simulink model "gm_RRCFilter"  (R2023b)
settings: Solver=FixedStepAuto  StartTime=0.0  StopTime=100.0  RelTol=1e-3  EnableMultiTasking=on
libraries: dspmlti4 x1, dspsrcs4 x1
settings Model: Creator=31651  LastModifiedBy=31651
settings SolverCC: PositivePriorityOrder=on
settings OptimizationCC: BlockReduction=off  ConditionallyExecuteInputs=off  EnhancedBackFolding=on  PassReuseOutputArgsAs=Individual arguments  ZeroExternalMemoryAtStartup=off  ZeroInternalMemoryAtStartup=off  MaxStackSize=64  OptimizeBlockOrder=speed  DifferentSizesBufferReuse=on  OptimizationCustomize=off  EfficientTunableParamExpr=on
settings DebuggingCC: InheritedTsInSrcMsg=none  SingleTaskRateTransMsg=error  ParameterPrecisionLossMsg=none  ParameterTunabilityLossMsg=error
settings HardwareCC: ProdBitPerPointer=32  ProdBitPerSizeT=32  ProdBitPerPtrDiffT=32  ProdLargestAtomicInteger=Long  ProdLargestAtomicFloat=Double  ProdWordSize=32  ProdHWDeviceType=ARM Compatible->ARM Cortex  HardwareBoardFeatureSet=SoCBlockset
settings ModelReferenceCC: ModelReferenceNumInstancesAllowed=Single
settings SFSimCC: MATLABDynamicMemAlloc=off
settings RTWCC: Description=Embedded Coder  SystemTargetFile=ert.tlc  HardwareBoard=ZedBoard  TLCOptions="-aInlineSetEventsForThisBaseRateFcn=TLC_FALSE -aSuppressMultiTaskScheduler=TLC_FALSE  -aRateBasedStepFcn=0"  TemplateMakefile=ert_default_tmf
settings CodeAppCC: ForceParamTrailComments=on  IgnoreCustomStorageClasses=off  OperatorAnnotations=on  SimulinkDataObjDesc=on  SFDataObjDesc=on  InsertBlockDesc=on

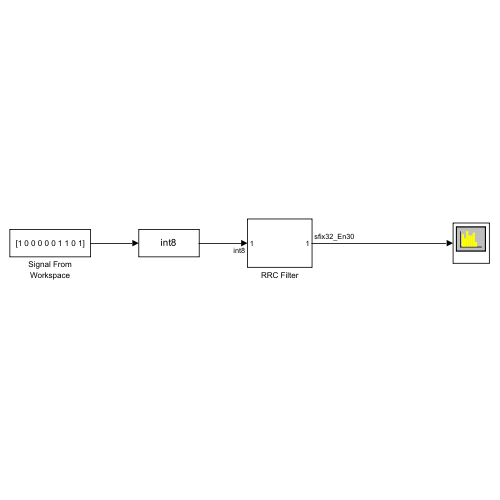
[thumbnail: Simulink's stored preview of the top-level diagram]
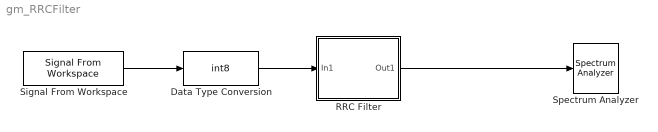
== system gm_RRCFilter ==
  Data Type Conversion : DataTypeConversion  OutDataTypeStr=int8  SaturateOnIntegerOverflow=off  RndMeth=Floor
  RRC Filter : Subsystem
  Signal From Workspace : dspsrcs4/Signal From Workspace  X=[1 0 0 0 0 0 1 1 0 1]  Ts=1  nsamps=1  OutputAfterFinalValue=Setting to zero  ignoreOrWarnInputAndFrameLengths=off  OutputFrames=off
  Spectrum Analyzer : SpectrumAnalyzer  WindowPosition=[560.000000,290.000000,800.000000,500.000000,]  Visible=on  ScopeFrameLocation=window  YLimits=[-1,1]
      settings: OpenAtSimulationStart=off
  wires:
  Data Type Conversion/1 -> RRC Filter/1(In1)
  RRC Filter/1(Out1) -> Spectrum Analyzer/1
  Signal From Workspace/1 -> Data Type Conversion/1

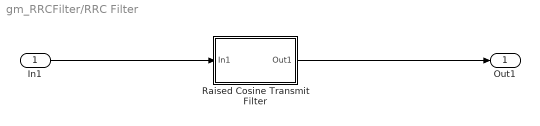
== system gm_RRCFilter/RRC Filter ==
  In1 : Inport  OutDataTypeStr=int8  PortDimensions=1  SampleTime=1
  Raised Cosine Transmit Filter : Subsystem  mask(Raised Cosine Transmit Filter){filtType=Square root, R=double(0.35), filtSpan=double(10), N=double(8), filterGain=double(1), InputProcessing=Elements as channels (sample based), RateOptions=Allow multirate processing, framing=Mute, checkCoeff=on, variableName=reshape(double([0.0026527855208223674 0.0011289546396784642 -0.0008407326480319395 -0.00276367829210128 -0.004110944765368385 -0.004461362499463928 -0.003631504382928873 -0.001754140268900142 0.0007223681197420734 0.0031229931857521803 0.004709784599647098 0.004885171607650034 0.0033846054323965124 0.0004047716742814459 -0.0033763672523499932 -0.006908879439330136 -0.00899992193184229 -0.008620760449754293 -0.005224208699525725 0.0010072932270158315 0.009056961535619827 0.01716189202348441 0.023104501384526945 0.024670913641949364 0.020196270831997543 0.009086336159429796 -0.007804452542466291 -0.028041986077568522 -0.047791391302472425 -0.06231040781338443 -0.06669696670055805 -0.056772614240839 -0.02994482367854878 0.014118459714553666 0.07314561775450068 0.14233999357591096 0.21489687901792265 0.2828943370509198 0.33842104994516803 0.37475541159859566 0.38739472380436457 0.37475541159859566 0.33842104994516803 0.2828943370509198 0.21489687901792265 0.14233999357591096 0.07314561775450068 0.014118459714553666 -0.02994482367854878 -0.056772614240839 -0.06669696670055805 -0.06231040781338443 -0.047791391302472425 -0.028041986077568522 -0.007804452542466291 0.009086336159429796 0.020196270831997543 0.024670913641949364 0.023104501384526945 0.01716189202348441 0.009056961535619827 0.0010072932270158315 -0.005224208699525725 -0.008620760449754293 -0.00899992193184229 -0.006908879439330136 -0.0033763672523499932 0.0004047716742814459 0.0033846054323965124 0.004885171607650034 0.004709784599647098 0.0031229931857521803 0.0007223681197420734 -0.001754140268900142 -0.003631504382928873 -0.004461362499463928 -0.004110944765368385 -0.00276367829210128 -0.0008407326480319395 0.0011289546396784642 0.0026527855208223674]).', [1  81]), checkGain=Normalized, sampMode=Mute, saveAsFlag=double(0), currentFiltSpan=double(10), D=double(5), launchFVT=on, roundingMode=Floor, overflowMode=off, coeffMode=Binary point scaling, coeffWordLength=double(32), coeffFracLength=double(30), coeffDataTypeStr=fixdt(1,32,30), coeffMin=[], coeffMax=[], coeffLastDataTypeStr=fixdt(1,32,30), prodOutputMode=Binary point scaling, prodOutputWordLength=double(32), prodOutputFracLength=double(30), prodOutputDataTypeStr=fixdt(1,32,30), prodOutputLastDataTypeStr=fixdt(1,32,30), accumMode=Binary point scaling, accumWordLength=double(32), accumFracLength=double(30), accumDataTypeStr=fixdt(1,32,30), accumLastDataTypeStr=fixdt(1,32,30), outputMode=Binary point scaling, outputWordLength=double(32), outputFracLength=double(30), outputDataTypeStr=fixdt(1,32,30), outputMin=[], outputMax=[], outputLastDataTypeStr=fixdt(1,32,30), LockScale=on}
      mask prompts: filtType "Filter shape:"; R "Rolloff factor:"; filtSpan "Filter span in symbols:"; N "Output samples per symbol:"; filterGain "Linear amplitude filter gain:"; InputProcessing "dsp:FIRMultirateBlockDialog:InputProc_MP"; RateOptions "dsp:FIRMultirateBlockDialog:RateOptions_MP"; checkCoeff "Export filter coefficients to workspace"; variableName "Coefficient variable name:"; checkGain "Filter gain:"; sampMode "Input sampling mode:"; saveAsFlag "Save_as flag:"; currentFiltSpan "Current filter span in symbols:"; D "Group delay (number of symbols):"; launchFVT "Visualize filter with FVTool"; roundingMode "dspshared:FixptDialog:roundingMode"; overflowMode "Simulink:masks:SaturateOnIntegerOverflow_MP"; LockScale "dspshared:FixptDialog:lockAgnstChanges"
      mask help: Upsample and filter the input signal using a normal or square root raised cosine FIR filter.
      mask init:
      | D = double(5);
      | InputProcessing = double(2);
      | LockScale = double(1);
      | N = double(8);
      | R = double(0.35);
      | RateOptions = double(2);
      | accumDataTypeStr = fixdt(1,32,30);
      | accumFracLength = double(30);
      | accumLastDataTypeStr = 'fixdt(1,32,30)';
      | accumMode = double(4);
      | accumWordLength = double(32);
      | checkCoeff = double(1);
      | checkGain = double(1);
      | coeff = reshape(double([0.0026527855208223674 0.0011289546396784642 -0.0008407326480319395 -0.00276367829210128 -0.004110944765368385 -0.004461362499463928 -0.003631504382928873 -0.001754140268900142 0.0007223681197420734 0.0031229931857521803 0.004709784599647098 0.004885171607650034 0.0033846054323965124 0.0004047716742814459 -0.0033763672523499932 -0.006908879439330136 -0.00899992193184229 -0.008620760449754293 -0.005224208699525725 0.0010072932270158315 0.009056961535619827 0.01716189202348441 0.023104501384526945 0.024670913641949364 0.020196270831997543 0.009086336159429796 -0.007804452542466291 -0.028041986077568522 -0.047791391302472425 -0.06231040781338443 -0.06669696670055805 -0.056772614240839 -0.02994482367854878 0.014118459714553666 0.07314561775450068 0.14233999357591096 0.21489687901792265 0.2828943370509198 0.33842104994516803 0.37475541159859566 0.38739472380436457 0.37475541159859566 0.33842104994516803 0.2828943370509198 0.21489687901792265 0.14233999357591096 0.07314561775450068 0.014118459714553666 -0.02994482367854878 -0.056772614240839 -0.06669696670055805 -0.06231040781338443 -0.047791391302472425 -0.028041986077568522 -0.007804452542466291 0.009086336159429796 0.020196270831997543 0.024670913641949364 0.023104501384526945 0.01716189202348441 0.009056961535619827 0.0010072932270158315 -0.005224208699525725 -0.008620760449754293 -0.00899992193184229 -0.006908879439330136 -0.0033763672523499932 0.0004047716742814459 0.0033846054323965124 0.004885171607650034 0.004709784599647098 0.0031229931857521803 0.0007223681197420734 -0.001754140268900142 -0.003631504382928873 -0.004461362499463928 -0.004110944765368385 -0.00276367829210128 -0.0008407326480319395 0.0011289546396784642 0.0026527855208223674]).', [1  81]);
      | coeffDataTypeStr = fixdt(1,32,30);
      | coeffFracLength = double(30);
      | coeffLastDataTypeStr = 'fixdt(1,32,30)';
      | coeffMax = [];
      | coeffMin = [];
      | coeffMode = double(3);
      | coeffWordLength = double(32);
      | currentFiltSpan = double(10);
      | filtSpan = double(10);
      | filtType = double(2);
      | filterGain = double(1);
      | framing = double(5);
      | launchFVT = double(1);
      | outputDataTypeStr = fixdt(1,32,30);
      | outputFracLength = double(30);
      | outputLastDataTypeStr = 'fixdt(1,32,30)';
      | outputMax = [];
      | outputMin = [];
      | outputMode = double(4);
      | outputWordLength = double(32);
      | overflowMode = double(0);
      | prodOutputDataTypeStr = fixdt(1,32,30);
      | prodOutputFracLength = double(30);
      | prodOutputLastDataTypeStr = 'fixdt(1,32,30)';
      | prodOutputMode = double(3);
      | prodOutputWordLength = double(32);
      | rateFactor = double(8);
      | roundingMode = double(3);
      | sampMode = double(3);
      | saveAsFlag = double(0);
      | variableName = 'rcTxFilt';
      mask Help: eval('blocksethelp');
      mask TypeOptions filtType: Normal | Square root
      mask TypeOptions InputProcessing: Columns as channels (frame based) | Elements as channels (sample based)
      mask Callback InputProcessing: commblkrcfilttx(gcbh,'cbInputProcessing');
      mask TypeOptions RateOptions: Enforce single-rate processing | Allow multirate processing
      mask TypeOptions framing: Enforce single-rate processing | Allow multirate processing | Maintain input frame rate | Maintain input frame size | Mute
      mask Callback checkCoeff: commblkrcfilttx(gcbh,'cbCheckCoeff');
      mask Callback variableName: commblkrcfilttx(gcbh,'dialogdynamic');
      mask TypeOptions checkGain: Normalized | User-specified
      mask TypeOptions sampMode: Frame-based | Sample-based | Mute
      mask TypeOptions roundingMode: Ceiling | Convergent | Floor | Nearest | Round | Simplest | Zero
      mask TypeOptions coeffMode: Same word length as input | Specify word length | Binary point scaling | Slope and bias scaling
      mask TypeOptions prodOutputMode: Inherit via internal rule | Same as input | Binary point scaling | Slope and bias scaling
      mask TypeOptions accumMode: Inherit via internal rule | Same as product output | Same as input | Binary point scaling | Slope and bias scaling
      mask TypeOptions outputMode: Same as accumulator | Same as product output | Same as input | Binary point scaling | Slope and bias scaling
      mask Display:
      | coeffs = rcosdesign(0.2, 10, 8, 'sqrt'); % default
      | % This plot does not change enough to make it worth updating to specifics
      | % Just use a representative plot for all cases.
      | %
      | %-- Init icon variables
      | %   (draw default icon in case of early returns,
      | %    e.g. due to errors from undefined mask params)
      | icon.str = get_param(gcbh,'filtType');
      | icon.x = 0.5;
      | icon.y = 0.25;
      | icon.plot = coeffs/max(coeffs)*0.40+0.50;
      | icon.xx = (1:length(coeffs))/length(coeffs);
      | 
      | plot(0,0,1,1,icon.xx,icon.plot);
      | text(icon.x,icon.y,icon.str,'horiz','center');
  Out1 : Outport  OutDataTypeStr=fixdt(1,32,30)  SampleTime=0.125
  wires:
  In1/1 -> Raised Cosine Transmit Filter/1(In1)
  Raised Cosine Transmit Filter/1(Out1) -> Out1/1

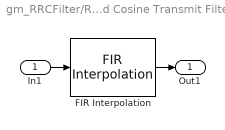
== system gm_RRCFilter/RRC Filter/Raised Cosine Transmit Filter ==
  In1 : Inport  OutDataTypeStr=int8  SampleTime=1
  FIR Interpolation : dspmlti4/FIR Interpolation  FilterSource=Dialog parameters  PrivateCoeffs=0  h=coeff  L=rateFactor  FilterObject=Hm_firinterp  framing=Allow multirate processing  outputBufInitCond=0  roundingMode=Floor  overflowMode=off  firstCoeffMode=Binary point scaling  firstCoeffWordLength=32  firstCoeffFracLength=30  firstCoeffDataTypeStr=fixdt(1,32,30)  firstCoeffMin=[]  firstCoeffMax=[]  firstCoeffLastDataTypeStr=fixdt(1,32,30)  prodOutputMode=Binary point scaling  prodOutputWordLength=32  prodOutputFracLength=30  prodOutputDataTypeStr=fixdt(1,32,30)  prodOutputLastDataTypeStr=fixdt(1,32,30)  accumMode=Binary point scaling  accumWordLength=32  accumFracLength=30  accumDataTypeStr=fixdt(1,32,30)  accumLastDataTypeStr=fixdt(1,32,30)  outputMode=Binary point scaling  outputWordLength=32  outputFracLength=30  outputDataTypeStr=fixdt(1,32,30)  outputMin=[]  outputMax=[]  outputLastDataTypeStr=fixdt(1,32,30)
      settings: LockScale=on
      settings: LibrarySourceBlock=|
      | commhdlfilt/Raised Cosine
      | Transmit Filter/FIR
      | Interpolation
  Out1 : Outport  SampleTime=0.125
  wires:
  In1/1 -> FIR Interpolation/1
  FIR Interpolation/1 -> Out1/1
